simulink library "xbsReplacements_r3"  (Simulink 5.1)
libraries: xbsIndex_r3 x22
settings Model: Creator=jballagh  LastModifiedBy=sps  ProdHWDeviceType=Microprocessor

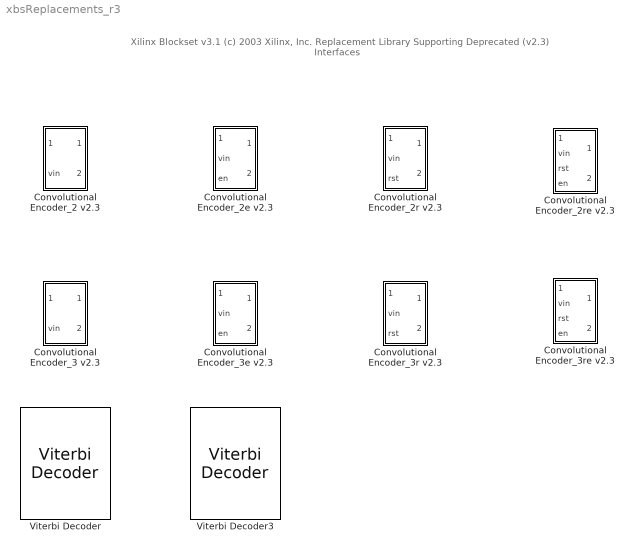
== system xbsReplacements_r3 ==
  note: Xilinx Blockset v3.1
      | (c) 2003 Xilinx, Inc.
      |
      | Replacement Library Supporting
      | Deprecated (v2.3) Interfaces
  Convolutional Encoder_2 v2.3 : Subsystem
  Convolutional Encoder_2e v2.3 : Subsystem  AncestorBlock=xbsReplacements_r3/Convolutional Encoder_2 v2.1
  Convolutional Encoder_2r v2.3 : Subsystem  AncestorBlock=xbsReplacements_r3/Convolutional Encoder_2 v2.3
  Convolutional Encoder_2re v2.3 : Subsystem  AncestorBlock=xbsReplacements_r3/Convolutional Encoder_2 v2.1
  Convolutional Encoder_3 v2.3 : Subsystem
  Convolutional Encoder_3e v2.3 : Subsystem  AncestorBlock=xbsReplacements_r3/Convolutional Encoder_3 v2.3
  Convolutional Encoder_3r v2.3 : Subsystem  AncestorBlock=xbsReplacements_r3/Convolutional Encoder_3 v2.3
  Convolutional Encoder_3re v2.3 : Subsystem  AncestorBlock=xbsReplacements_r3/Convolutional Encoder_3 v2.3
  Viterbi Decoder : xbsIndex_r3/Viterbi Decoder  clength=7  dual_decoding=off  conv_codes=[117 127]  conv_codes2=[117 127]  tb_length=100  coding=Hard  data_format=Signed Magnitude  architecture=Parallel  optimization=Area  puncturing=off  best_state=off  best_state_wr=0  red_latency=off  explicit_period=off  period=1  has_ber=off  ber_rate=20  has_norm=off  rst=off  en=off  dbl_ovrd=off  use_rpm=on  gen_core=on
      settings: xl_area=[0, 0, 0, 0, 0, 0, 0]
  Viterbi Decoder3 : xbsIndex_r3/Viterbi Decoder  clength=7  dual_decoding=off  conv_codes=[117 127 135]  conv_codes2=[117 127]  tb_length=100  coding=Hard  data_format=Signed Magnitude  architecture=Parallel  optimization=Area  puncturing=off  best_state=off  best_state_wr=0  red_latency=off  explicit_period=off  period=1  has_ber=off  ber_rate=20  has_norm=off  rst=off  en=off  dbl_ovrd=off  use_rpm=on  gen_core=on
      settings: xl_area=[0, 0, 0, 0, 0, 0, 0]

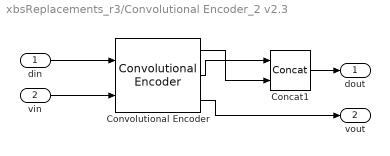
== system xbsReplacements_r3/Convolutional Encoder_2 v2.3 ==
  din : Inport
  vin : Inport  Port=2
  Concat1 : xbsIndex_r3/Concat  explicit_period=off  period=1  dbl_ovrd=off
  Convolutional Encoder : xbsIndex_r3/Convolutional Encoder  clength=3  conv_codes=[7 5]  explicit_period=off  period=1  rst=off  en=off  dbl_ovrd=off  gen_core=on  use_rpm=on
      settings: xl_area=[0, 0, 0, 0, 0, 0, 0]
  dout : Outport
  vout : Outport  Port=2
  wires:
  Convolutional Encoder/1 -> Concat1/2
  Convolutional Encoder/2 -> Concat1/1
  Convolutional Encoder/3 -> vout/1
  Concat1/1 -> dout/1
  vin/1 -> Convolutional Encoder/2
  din/1 -> Convolutional Encoder/1

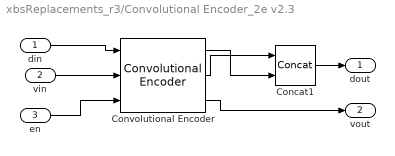
== system xbsReplacements_r3/Convolutional Encoder_2e v2.3 ==
  din : Inport
  vin : Inport  Port=2
  en : Inport  Port=3
  Concat1 : xbsIndex_r3/Concat  explicit_period=off  period=1  dbl_ovrd=off
  Convolutional Encoder : xbsIndex_r3/Convolutional Encoder  clength=3  conv_codes=[7 5]  explicit_period=off  period=1  rst=off  en=on  dbl_ovrd=off  gen_core=on  use_rpm=on
      settings: xl_area=[0, 0, 0, 0, 0, 0, 0]
  dout : Outport
  vout : Outport  Port=2
  wires:
  Convolutional Encoder/1 -> Concat1/2
  Convolutional Encoder/2 -> Concat1/1
  Convolutional Encoder/3 -> vout/1
  Concat1/1 -> dout/1
  vin/1 -> Convolutional Encoder/2
  din/1 -> Convolutional Encoder/1
  en/1 -> Convolutional Encoder/3

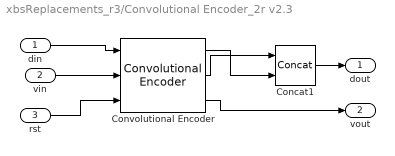
== system xbsReplacements_r3/Convolutional Encoder_2r v2.3 ==
  din : Inport
  vin : Inport  Port=2
  rst : Inport  Port=3
  Concat1 : xbsIndex_r3/Concat  explicit_period=off  period=1  dbl_ovrd=off
  Convolutional Encoder : xbsIndex_r3/Convolutional Encoder  clength=3  conv_codes=[7 5]  explicit_period=off  period=1  rst=on  en=off  dbl_ovrd=off  gen_core=on  use_rpm=on
      settings: xl_area=[0, 0, 0, 0, 0, 0, 0]
  dout : Outport
  vout : Outport  Port=2
  wires:
  Convolutional Encoder/1 -> Concat1/2
  Convolutional Encoder/2 -> Concat1/1
  Convolutional Encoder/3 -> vout/1
  Concat1/1 -> dout/1
  vin/1 -> Convolutional Encoder/2
  din/1 -> Convolutional Encoder/1
  rst/1 -> Convolutional Encoder/3

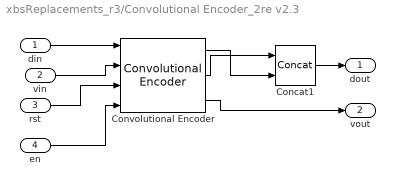
== system xbsReplacements_r3/Convolutional Encoder_2re v2.3 ==
  din : Inport
  vin : Inport  Port=2
  rst : Inport  Port=3
  en : Inport  Port=4
  Concat1 : xbsIndex_r3/Concat  explicit_period=off  period=1  dbl_ovrd=off
  Convolutional Encoder : xbsIndex_r3/Convolutional Encoder  clength=3  conv_codes=[7 5]  explicit_period=off  period=1  rst=on  en=on  dbl_ovrd=off  gen_core=on  use_rpm=on
      settings: xl_area=[0, 0, 0, 0, 0, 0, 0]
  dout : Outport
  vout : Outport  Port=2
  wires:
  Convolutional Encoder/1 -> Concat1/2
  Convolutional Encoder/2 -> Concat1/1
  Convolutional Encoder/3 -> vout/1
  Concat1/1 -> dout/1
  vin/1 -> Convolutional Encoder/2
  din/1 -> Convolutional Encoder/1
  rst/1 -> Convolutional Encoder/3
  en/1 -> Convolutional Encoder/4

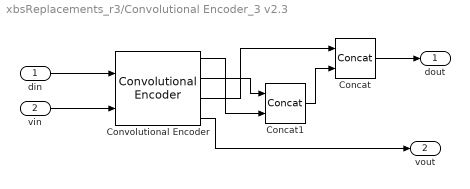
== system xbsReplacements_r3/Convolutional Encoder_3 v2.3 ==
  din : Inport
  vin : Inport  Port=2
  Concat : xbsIndex_r3/Concat  explicit_period=off  period=1  dbl_ovrd=off
      settings: xl_area=[0, 0, 0, 0, 0, 0, 0]
  Concat1 : xbsIndex_r3/Concat  explicit_period=off  period=1  dbl_ovrd=off
      settings: xl_area=[0, 0, 0, 0, 0, 0, 0]
  Convolutional Encoder : xbsIndex_r3/Convolutional Encoder  clength=3  conv_codes=[7 5 6]  explicit_period=off  period=1  rst=off  en=off  dbl_ovrd=off  gen_core=on  use_rpm=on
      settings: xl_area=[0, 0, 0, 0, 0, 0, 0]
  dout : Outport
  vout : Outport  Port=2
  wires:
  Convolutional Encoder/1 -> Concat1/2
  Convolutional Encoder/2 -> Concat1/1
  Concat1/1 -> Concat/2
  Convolutional Encoder/3 -> Concat/1
  Convolutional Encoder/4 -> vout/1
  Concat/1 -> dout/1
  vin/1 -> Convolutional Encoder/2
  din/1 -> Convolutional Encoder/1

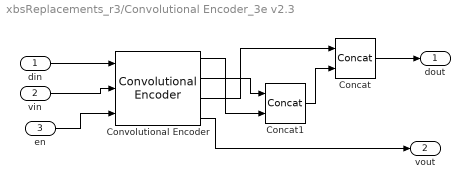
== system xbsReplacements_r3/Convolutional Encoder_3e v2.3 ==
  din : Inport
  vin : Inport  Port=2
  en : Inport  Port=3
  Concat : xbsIndex_r3/Concat  explicit_period=off  period=1  dbl_ovrd=off
  Concat1 : xbsIndex_r3/Concat  explicit_period=off  period=1  dbl_ovrd=off
  Convolutional Encoder : xbsIndex_r3/Convolutional Encoder  clength=3  conv_codes=[7 5 6]  explicit_period=off  period=1  rst=off  en=on  dbl_ovrd=off  gen_core=on  use_rpm=on
      settings: xl_area=[0, 0, 0, 0, 0, 0, 0]
  dout : Outport
  vout : Outport  Port=2
  wires:
  Convolutional Encoder/1 -> Concat1/2
  Convolutional Encoder/2 -> Concat1/1
  Concat1/1 -> Concat/2
  Convolutional Encoder/3 -> Concat/1
  Convolutional Encoder/4 -> vout/1
  Concat/1 -> dout/1
  vin/1 -> Convolutional Encoder/2
  din/1 -> Convolutional Encoder/1
  en/1 -> Convolutional Encoder/3

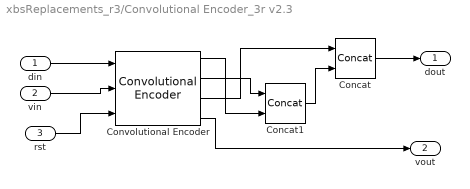
== system xbsReplacements_r3/Convolutional Encoder_3r v2.3 ==
  din : Inport
  vin : Inport  Port=2
  rst : Inport  Port=3
  Concat : xbsIndex_r3/Concat  explicit_period=off  period=1  dbl_ovrd=off
  Concat1 : xbsIndex_r3/Concat  explicit_period=off  period=1  dbl_ovrd=off
  Convolutional Encoder : xbsIndex_r3/Convolutional Encoder  clength=3  conv_codes=[7 5 6]  explicit_period=off  period=1  rst=on  en=off  dbl_ovrd=off  gen_core=on  use_rpm=on
      settings: xl_area=[0, 0, 0, 0, 0, 0, 0]
  dout : Outport
  vout : Outport  Port=2
  wires:
  Convolutional Encoder/1 -> Concat1/2
  Convolutional Encoder/2 -> Concat1/1
  Concat1/1 -> Concat/2
  Convolutional Encoder/3 -> Concat/1
  Convolutional Encoder/4 -> vout/1
  Concat/1 -> dout/1
  vin/1 -> Convolutional Encoder/2
  din/1 -> Convolutional Encoder/1
  rst/1 -> Convolutional Encoder/3

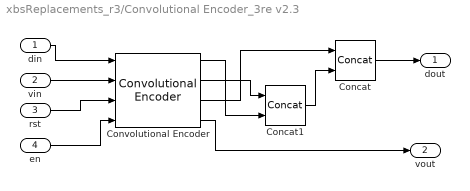
== system xbsReplacements_r3/Convolutional Encoder_3re v2.3 ==
  din : Inport
  vin : Inport  Port=2
  rst : Inport  Port=3
  en : Inport  Port=4
  Concat : xbsIndex_r3/Concat  explicit_period=off  period=1  dbl_ovrd=off
  Concat1 : xbsIndex_r3/Concat  explicit_period=off  period=1  dbl_ovrd=off
  Convolutional Encoder : xbsIndex_r3/Convolutional Encoder  clength=3  conv_codes=[7 5 6]  explicit_period=off  period=1  rst=on  en=on  dbl_ovrd=off  gen_core=on  use_rpm=on
      settings: xl_area=[0, 0, 0, 0, 0, 0, 0]
  dout : Outport
  vout : Outport  Port=2
  wires:
  Convolutional Encoder/1 -> Concat1/2
  Convolutional Encoder/2 -> Concat1/1
  Concat1/1 -> Concat/2
  Convolutional Encoder/3 -> Concat/1
  Convolutional Encoder/4 -> vout/1
  Concat/1 -> dout/1
  vin/1 -> Convolutional Encoder/2
  din/1 -> Convolutional Encoder/1
  rst/1 -> Convolutional Encoder/3
  en/1 -> Convolutional Encoder/4
